simulink model "obs_com_filtro_2014"  (R2014b)
settings: Solver=ode45  SolverMode=SingleTasking  StartTime=0.0  StopTime=600  RelTol=1e-3
model workspace (MAT data in the model file):
  Td = 2
  std_dev = 0.08
values from neighbouring files (symbols this model uses):
  K = 0.002677    [run_and_calculate.m]
  T = 0.5    [run_and_calculate.m]
undefined symbols (not defined in the file): sigma_n
libraries: cstblocks x27
(part 2 of 2)

== matlab function obs_com_filtro_2014/Statistic Filter7 ==
  settings: updateMethod=DISCRETE
  data: u input; saida_filtro output; std_dev parameter; alpha output
%Autor: Lucas Moura Gomes
%Filtro estatístico.

function [saida_filtro, alpha]  = filtroPID( u, std_dev)
    persistent x_ant;
    persistent alpha_orig;
    
    if isempty(x_ant)
        x_ant = 0;
        Ts = 0.01; %sampling time
        tf = 2; %continuous time cte.
        alpha_orig = 1 - exp(-1/tf * Ts); %c2d filter
    end
    
    alpha = erf(abs(x_ant - u)/(sqrt(2)*2*std_dev));
    
    if alpha > 1
        alpha = 1;
    end
    
    %up = 1.1; %upper bound 10%
    %alpha = alpha * alpha_orig * up;
    
    saida_filtro = (1-alpha)*x_ant + alpha*u;
    
    x_ant = saida_filtro;
end

%Autor: Lucas Moura Gomes
%Filtro estatístico.
% 
% function [saida_filtro, alpha] = filtroPID( u, erro_tipico_medicao, Tf  )
% 	
%     persistent x_ant;
%     
%     if isempty(x_ant)
%         x_ant = 0;
%     end
%     
%     Tf = Tf/1.5;
%     a_Tf = 1 - exp(-1/Tf * 5);
%     
%     alpha = erf(abs(x_ant - u)/(sqrt(2)*2*erro_tipico_medicao));
%     
%     if alpha > 1 
%         alpha = 1;
%     end;
%     
%     saida_filtro = (1-alpha)*x_ant + alpha*u;
% 
%     x_ant = saida_filtro;
%         
% 
%     saida_filtro = x_ant;
% 
%     
% end

== matlab function obs_com_filtro_2014/Statistic Filter8 ==
  settings: updateMethod=DISCRETE
  data: u input; saida_filtro output; std_dev parameter; alpha output
%Autor: Lucas Moura Gomes
%Filtro estatístico.

function [saida_filtro, alpha]  = filtroPID( u, std_dev)
    persistent x_ant;
    persistent alpha_orig;
    
    if isempty(x_ant)
        x_ant = 0;
        Ts = 0.01; %sampling time
        tf = 2; %continuous time cte.
        alpha_orig = 1 - exp(-1/tf * Ts); %c2d filter
    end
    
    alpha = erf(abs(x_ant - u)/(sqrt(2)*2*std_dev));
    
    if alpha > 1
        alpha = 1;
    end
    
    %up = 1.1; %upper bound 10%
    %alpha = alpha * alpha_orig * up;
    
    saida_filtro = (1-alpha)*x_ant + alpha*u;
    
    x_ant = saida_filtro;
end

%Autor: Lucas Moura Gomes
%Filtro estatístico.
% 
% function [saida_filtro, alpha] = filtroPID( u, erro_tipico_medicao, Tf  )
% 	
%     persistent x_ant;
%     
%     if isempty(x_ant)
%         x_ant = 0;
%     end
%     
%     Tf = Tf/1.5;
%     a_Tf = 1 - exp(-1/Tf * 5);
%     
%     alpha = erf(abs(x_ant - u)/(sqrt(2)*2*erro_tipico_medicao));
%     
%     if alpha > 1 
%         alpha = 1;
%     end;
%     
%     saida_filtro = (1-alpha)*x_ant + alpha*u;
% 
%     x_ant = saida_filtro;
%         
% 
%     saida_filtro = x_ant;
% 
%     
% end

== matlab function obs_com_filtro_2014/Statistic Filter9 ==
  settings: updateMethod=DISCRETE
  data: u input; saida_filtro output; std_dev parameter; alpha output
%Autor: Lucas Moura Gomes
%Filtro estatístico.

function [saida_filtro, alpha]  = filtroPID( u, std_dev)
    persistent x_ant;
    persistent alpha_orig;
    
    if isempty(x_ant)
        x_ant = 0;
        Ts = 0.01; %sampling time
        tf = 2; %continuous time cte.
        alpha_orig = 1 - exp(-1/tf * Ts); %c2d filter
    end
    
    alpha = erf(abs(x_ant - u)/(sqrt(2)*2*std_dev));
    
    if alpha > 1
        alpha = 1;
    end
    
    %up = 1.1; %upper bound 10%
    %alpha = alpha * alpha_orig * up;
    
    saida_filtro = (1-alpha)*x_ant + alpha*u;
    
    x_ant = saida_filtro;
end

%Autor: Lucas Moura Gomes
%Filtro estatístico.
% 
% function [saida_filtro, alpha] = filtroPID( u, erro_tipico_medicao, Tf  )
% 	
%     persistent x_ant;
%     
%     if isempty(x_ant)
%         x_ant = 0;
%     end
%     
%     Tf = Tf/1.5;
%     a_Tf = 1 - exp(-1/Tf * 5);
%     
%     alpha = erf(abs(x_ant - u)/(sqrt(2)*2*erro_tipico_medicao));
%     
%     if alpha > 1 
%         alpha = 1;
%     end;
%     
%     saida_filtro = (1-alpha)*x_ant + alpha*u;
% 
%     x_ant = saida_filtro;
%         
% 
%     saida_filtro = x_ant;
% 
%     
% end
